simulink model "CtrlP"  (R2019b)
settings: Solver=FixedStepAuto  StartTime=0.0  StopTime=inf  FixedStep=0.002  RelTol=1e-3
model workspace (MAT data in the model file):
  SL_ROS_VariableLengthArrays_MaxSizes.CommonInfo.ArrayTruncateAction = 'EmitWarning'
  SL_ROS_VariableLengthArrays_MaxSizes.MsgTypeMap = containers.Map
  SL_ROS_VariableLengthArrays_MaxSizes.MsgTypeMap.serialization.keys = {'std_msgs/Float64MultiArray'}
  SL_ROS_VariableLengthArrays_MaxSizes.MsgTypeMap.serialization.values{1}.PropertyName = 'Data'
  SL_ROS_VariableLengthArrays_MaxSizes.MsgTypeMap.serialization.values{1}.DataType = 'double'
  SL_ROS_VariableLengthArrays_MaxSizes.MsgTypeMap.serialization.values{1}.MaxLength = 2
  SL_ROS_VariableLengthArrays_MaxSizes.MsgTypeMap.serialization.uniformity = 0
  SL_ROS_VariableLengthArrays_MaxSizes.MsgTypeMap.serialization.keyType = 'char'
  SL_ROS_VariableLengthArrays_MaxSizes.MsgTypeMap.serialization.valueType = 'any'
undefined symbols (not defined in the file or in its folder): Data, Data_SL_Info
libraries: robotlib x3
settings Model: Creator=anie  LastModifiedBy=anie
settings OptimizationCC: EnhancedBackFolding=on  PassReuseOutputArgsAs=Individual arguments  ZeroExternalMemoryAtStartup=off  ZeroInternalMemoryAtStartup=off  MaxStackSize=64  OptimizeBlockOrder=speed  DifferentSizesBufferReuse=on  OptimizationCustomize=off  EfficientTunableParamExpr=on
settings DebuggingCC: ParameterTunabilityLossMsg=error
settings HardwareCC: ProdBitPerLong=64  ProdHWDeviceType=Intel->x86-64 (Linux 64)
settings RTWCC: SystemTargetFile=ert.tlc  HardwareBoard=Robot Operating System (ROS)  TLCOptions="-aInlineSetEventsForThisBaseRateFcn=TLC_FALSE -aSuppressMultiTaskScheduler=TLC_FALSE  -aRateBasedStepFcn=0"  TemplateMakefile=ert_default_tmf  GenerateReport=on  Toolchain=Catkin  IncludeHyperlinkInReport=on  LaunchReport=on  TargetLang=C++  GenerateTraceInfo=on  GenerateTraceReport=on  GenerateTraceReportSl=on  GenerateTraceReportSf=on  GenerateTraceReportEml=on
settings CodeAppCC: ForceParamTrailComments=on  IgnoreCustomStorageClasses=off  OperatorAnnotations=on  SimulinkDataObjDesc=on  SFDataObjDesc=on  InsertBlockDesc=on

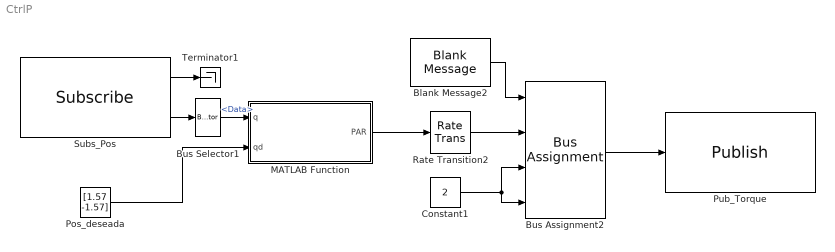
== system CtrlP ==
  Blank Message2 : robotlib/Blank Message  messageClass=Message  entityType=std_msgs/Float64MultiArray  messageType=std_msgs/Float64MultiArray  SampleTime=0.002
      settings: SourceProductName=ROS Toolbox
  Bus Assignment2 : BusAssignment  AssignedSignals=Data,Data_SL_Info.CurrentLength,Data_SL_Info.ReceivedLength
  Bus Selector1 : BusSelector  OutputSignals=Data
  Constant1 : Constant  Value=2  OutDataTypeStr=uint32  SampleTime=0.002
  MATLAB Function : MATLAB Function  TreatAsAtomicUnit=on
  Pos_deseada : Constant  Value=[1.57 -1.57]
  Pub_Torque : robotlib/Publish  topicSource=Specify your own  topic=/torque  messageType=std_msgs/Float64MultiArray  messageQueueLength=1
      settings: SourceProductName=ROS Toolbox
  Rate Transition2 : RateTransition
  Subs_Pos : robotlib/Subscribe  topicSource=Specify your own  topic=/pos  messageType=std_msgs/Float64MultiArray  sampleTime=-1  messageQueueLength=1
      settings: SourceProductName=ROS Toolbox
  Terminator1 : Terminator
  wires:
  Subs_Pos/1 -> Terminator1/1
  Pos_deseada/1 -> MATLAB Function/2(qd)
  Rate Transition2/1 -> Bus Assignment2/2
  Blank Message2/1 -> Bus Assignment2/1
  Constant1/1 -> Bus Assignment2/3, Bus Assignment2/4
  Subs_Pos/2 -> Bus Selector1/1
  Bus Assignment2/1 -> Pub_Torque/1
  Bus Selector1/1 -> MATLAB Function/1(q)  "<Data>"
  MATLAB Function/1(PAR) -> Rate Transition2/1

== matlab function CtrlP/MATLAB Function ==
  data: q input; qd input; PAR output
function PAR   = CTRLPDG(q,qd)

tau = [0 0];
T = 0.005;
n = 2;

kp = [10 10];
%kd = [0 0];
E = [0 0];
dotE = [0 0];
%intE(i) = [0 0]
Eant = [0 0];
    for i = 1:n
        E(i) = q(i) - qd(i);
        dotE(i) = (E(i) - Eant(i))/T;
        %intE(i) = E(i) * T;
        Eant(i) = E(i);
    end
    for i = 1:n
        tau(i) = -kp(i)*E(i);
        %tau(i) = - kp(i)*E(i) - kd(i)*dotE(i); % Par
        %tau(i) = - kp_PID(i)*E(i) - ki_PID(i)*intE(i) - kd_PID(i)*dotE(i); % Par
    end
PAR = tau;
